simulink library "localApparentWind_ul"  (R2018b)
settings: Solver=VariableStepAuto  StartTime=0.0  StopTime=10.0  RelTol=1e-3
libraries: vrlib x1
settings Model: Creator=mcobb  LastModifiedBy=mcobb

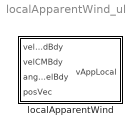
== system localApparentWind_ul ==
  localApparentWind : Subsystem

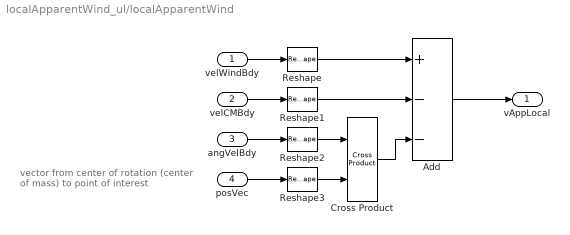
== system localApparentWind_ul/localApparentWind ==
  note: vector from center of rotation
      | (center of mass) to point of interest
  velWindBdy : Inport
  velCMBdy : Inport  Port=2
  angVelBdy : Inport  Port=3
  posVec : Inport  Port=4
  Add : Sum  Inputs=+--
  Cross Product : vrlib/Utilities/Cross Product
      settings: SourceProductBaseCode=VR
  Reshape{,1..3} (4 alike) : Reshape  OutputDimensionality=Column vector (2-D)
  vAppLocal : Outport
  wires:
  Cross Product/1 -> Add/3
  velWindBdy/1 -> Reshape/1
  velCMBdy/1 -> Reshape1/1
  angVelBdy/1 -> Reshape2/1
  posVec/1 -> Reshape3/1
  Reshape3/1 -> Cross Product/2
  Reshape2/1 -> Cross Product/1
  Reshape1/1 -> Add/2
  Reshape/1 -> Add/1
  Add/1 -> vAppLocal/1
